simulink model "WS_3DRobot_example_V2"  (R2023a)
settings: Solver=ode2  StartTime=0.0  StopTime=tsim  FixedStep=t_sample  RelTol=1e-3
values from neighbouring files (symbols this model uses):
  initialConfig = homeConfiguration(robot)    [Indy4_Matlab_Robo_Code.m]    (also in simout.mat = [0 0 0 0 0 0])
  Kd1 = 10    [Indy4_Matlab_Robo_Code.m]    (also in simout.mat)
  Kd2 = 10    [Indy4_Matlab_Robo_Code.m]    (also in simout.mat)
  Kd3 = 10    [Indy4_Matlab_Robo_Code.m]    (also in simout.mat)
  Kfilt1 = 150    [Indy4_Matlab_Robo_Code.m]    (also in simout.mat)
  Kfilt2 = 150    [Indy4_Matlab_Robo_Code.m]    (also in simout.mat)
  Kfilt3 = 150    [Indy4_Matlab_Robo_Code.m]    (also in simout.mat)
  Kp1 = 100    [Indy4_Matlab_Robo_Code.m]    (also in simout.mat)
  Kp2 = 100    [Indy4_Matlab_Robo_Code.m]    (also in simout.mat)
  Kp3 = 100    [Indy4_Matlab_Robo_Code.m]    (also in simout.mat)
undefined symbols (not defined in the file or in its folder): ctrlLowerLimit, ctrlUpperLimit, eePos_des_sim, eul2tform
libraries: robotmaniplib x6, robotcorelib x4, slpidlib x3
settings Model: Creator=ha281  LastModifiedBy=james
settings SolverCC: AlgebraicLoopSolver=TrustRegion
settings DataIOCC: ReturnWorkspaceOutputs=off
settings DebuggingCC: UnconnectedInputMsg=warning  UnconnectedOutputMsg=warning  UnconnectedLineMsg=warning  ArithmeticOperatorsInVariantConditions=warning
settings ModelReferenceCC: EnableRefExpFcnMdlSchedulingChecks=on
settings SFSimCC: SimUseLocalCustomCode=off  CustomCodeUndefinedFunction=UseInterfaceOnly
settings RTWCC: RTWUseLocalCustomCode=off
settings CodeAppCC: StateflowObjectComments=on

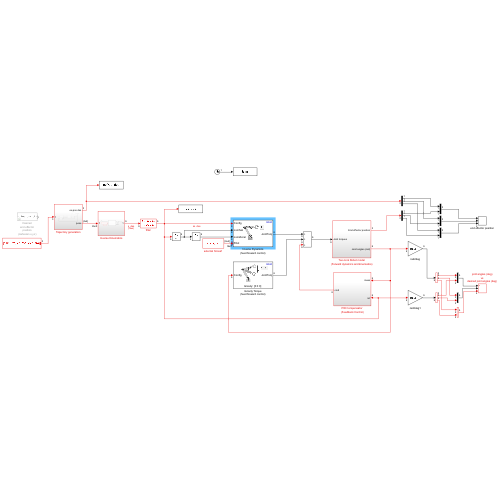
[thumbnail: Simulink's stored preview of the top-level diagram]
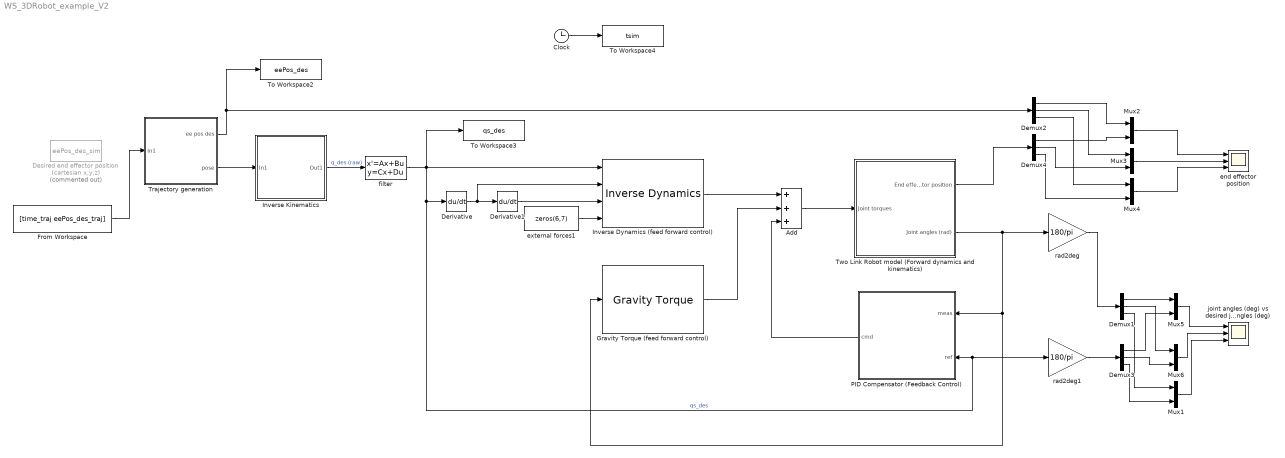
== system WS_3DRobot_example_V2 ==
  Add : Sum  Inputs=+++
  Clock : Clock
  Demux{1..4} (4 alike) : Demux  Outputs=3
  Derivative : Derivative
  Derivative1 : Derivative
  Desired end effector position (cartesian x,y,z) : Constant  Commented=on  Value=eePos_des_sim
  From Workspace : FromWorkspace  VariableName=[time_traj eePos_des_traj]
  Gravity Torque (feed forward control) : robotmaniplib/Gravity Torque  RigidBodyTree=robot  SimulateUsing=Interpreted execution
  Inverse Dynamics (feed forward control) : robotmaniplib/Inverse Dynamics  RigidBodyTree=robot  SimulateUsing=Interpreted execution
  Inverse Kinematics : Subsystem
  Mux{1..6} (6 alike) : Mux  Inputs=2
  PID Compensator (Feedback Control) : Subsystem
  To Workspace2 : ToWorkspace  VariableName=eePos_des  SampleTime=-1
  To Workspace3 : ToWorkspace  VariableName=qs_des  SampleTime=-1
  To Workspace4 : ToWorkspace  VariableName=tsim  SampleTime=-1
  Trajectory generation : Subsystem
  Two Link Robot model (Forward dynamics and kinematics) : Subsystem
  end effector position : Scope  NumInputPorts=3
  external forces1 : Constant  Value=zeros(6,7)
  filter : StateSpace  A=-1*eye(6)  B=1*eye(6)  C=eye(6)  D=zeros(6,6)  InitialCondition=0
  joint angles (deg) vs desired joint angles (deg) : Scope  NumInputPorts=3
  rad2deg : Gain  Gain=180/pi
  rad2deg1 : Gain  Gain=180/pi
  wires:
  Clock/1 -> To Workspace4/1
  rad2deg/1 -> Demux1/1
  Two Link Robot model (Forward dynamics and kinematics)/2(Joint angles (rad)) -> Gravity Torque (feed forward control)/1, PID Compensator (Feedback Control)/1(meas), rad2deg/1
  Derivative/1 -> Inverse Dynamics (feed forward control)/2, Derivative1/1
  Derivative1/1 -> Inverse Dynamics (feed forward control)/3
  external forces1/1 -> Inverse Dynamics (feed forward control)/4
  Inverse Dynamics (feed forward control)/1 -> Add/1
  Gravity Torque (feed forward control)/1 -> Add/2
  Add/1 -> Two Link Robot model (Forward dynamics and kinematics)/1(Joint torques)
  PID Compensator (Feedback Control)/1(cmd) -> Add/3
  Demux1/1 -> Mux5/1
  Demux3/2 -> Mux6/2
  Mux5/1 -> joint angles (deg) vs desired joint angles (deg)/1
  Demux3/1 -> Mux5/2
  Demux1/2 -> Mux6/1
  Mux6/1 -> joint angles (deg) vs desired joint angles (deg)/2
  rad2deg1/1 -> Demux3/1
  filter/1 -> To Workspace3/1, rad2deg1/1, PID Compensator (Feedback Control)/2(ref), Derivative/1, Inverse Dynamics (feed forward control)/1  "qs_des"
  Inverse Kinematics/1(Out1) -> filter/1  "q_des (raw)"
  Trajectory generation/2(pose) -> Inverse Kinematics/1(In1)
  Demux2/3 -> Mux4/1
  Trajectory generation/1(ee pos des) -> To Workspace2/1, Demux2/1
  Mux4/1 -> end effector position/3
  Demux4/3 -> Mux4/2
  Two Link Robot model (Forward dynamics and kinematics)/1(End effector position) -> Demux4/1
  Demux2/2 -> Mux3/1
  Mux3/1 -> end effector position/2
  Demux4/1 -> Mux2/2
  Mux2/1 -> end effector position/1
  Demux4/2 -> Mux3/2
  Demux2/1 -> Mux2/1
  From Workspace/1 -> Trajectory generation/1(In1)
  Demux1/3 -> Mux1/1
  Demux3/3 -> Mux1/2
  Mux1/1 -> joint angles (deg) vs desired joint angles (deg)/3

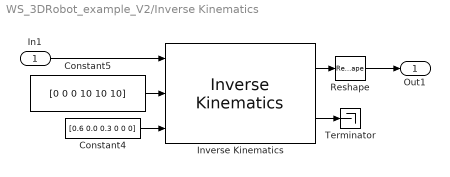
== system WS_3DRobot_example_V2/Inverse Kinematics ==
  In1 : Inport
  Constant4 : Constant  Value=[0.6 0.0 0.3 0 0 0]
  Constant5 : Constant  Value=[0 0 0 10 10 10]
  Inverse Kinematics : robotmaniplib/Inverse Kinematics  RigidBodyTree=robot  EndEffector=tool  ShowInfo=on  SolverName=BFGS Gradient Projection  EnforceJointLimits=on  MaxIterations=1500  MaxTime=10  GradientTolerance=1e-7  SolutionTolerance=1e-6  StepTolerance=1e-14  ErrorChangeTolerance=1e-12  UseErrorDamping=on  DampingBias=0.0025  SimulateUsing=Interpreted execution
  Reshape : Reshape
  Terminator : Terminator
  Out1 : Outport
  wires:
  Constant5/1 -> Inverse Kinematics/2
  Inverse Kinematics/2 -> Terminator/1
  Inverse Kinematics/1 -> Reshape/1
  Constant4/1 -> Inverse Kinematics/3
  Reshape/1 -> Out1/1
  In1/1 -> Inverse Kinematics/1

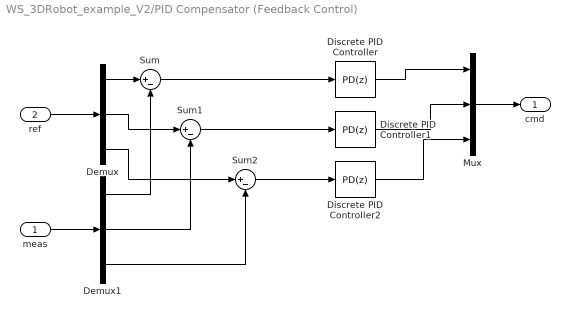
== system WS_3DRobot_example_V2/PID Compensator (Feedback Control) ==
  meas : Inport
  ref : Inport  Port=2
  Demux : Demux  Outputs=3
  Demux1 : Demux  Outputs=3
  Discrete PID Controller : slpidlib/PID Controller  Controller=PD  Form=Parallel  TimeDomain=Discrete-time  UseExternalTs=off  SampleTime=-1  IntegratorMethod=Forward Euler  FilterMethod=Forward Euler  ControllerParametersSource=internal  P=Kp1  I=0.01  UseKiTs=off  D=Kd1  N=Kfilt1  UseFilter=on  TunerSelectOption=Transfer Function Based (PID Tuner App)  InitialConditionSource=internal  InitialConditionForIntegrator=0  InitialConditionForFilter=0  DifferentiatorICPrevScaledInput=0  ExternalReset=none  TrackingMode=off  Kt=1  LimitOutput=off  SatLimitsSource=internal  UpperSaturationLimit=ctrlUpperLimit  LowerSaturationLimit=ctrlLowerLimit  LinearizeAsGain=off  AntiWindupMode=clamping  Kb=1  LimitIntegrator=off  UpperIntegratorSaturationLimit=inf  LowerIntegratorSaturationLimit=-inf  POutMin=[]  POutMax=[]  IOutMin=[]  IOutMax=[]  DOutMin=[]  DOutMax=[]  NOutMin=[]  NOutMax=[]  SumOutMin=[]  SumOutMax=[]  SaturationOutMin=[]  SaturationOutMax=[]  PParamMin=[]  PParamMax=[]  IParamMin=[]  IParamMax=[]  DParamMin=[]  DParamMax=[]  NParamMin=[]  NParamMax=[]  KbParamMin=[]  KbParamMax=[]  KtParamMin=[]  KtParamMax=[]  KbOutMin=[]  KbOutMax=[]  KtOutMin=[]  KtOutMax=[]  IntegratorOutMin=[]  IntegratorOutMax=[]  FilterOutMin=[]  FilterOutMax=[]  SumI1OutMin=[]  SumI1OutMax=[]  SumI2OutMin=[]  SumI2OutMax=[]  SumI3OutMin=[]  SumI3OutMax=[]  SumI4OutMin=[]  SumI4OutMax=[]  SumDOutMin=[]  SumDOutMax=[]  DifferentiatorOutMin=[]  DifferentiatorOutMax=[]  FilterDiffOutCoefMin=[]  FilterDiffOutCoefMax=[]  ReciprocalOutMin=[]  ReciprocalOutMax=[]  SumDenOutMin=[]  SumDenOutMax=[]  SumNumOutMin=[]  SumNumOutMax=[]  DivideOutMin=[]  DivideOutMax=[]  UdiffTsProdOutMin=[]  UdiffTsProdOutMax=[]  NTsProdOutMin=[]  NTsProdOutMax=[]  UintegralTsProdOutMin=[]  UintegralTsProdOutMax=[]  UngainTsProdOutMin=[]  UngainTsProdOutMax=[]  ClampingZeroOutDataTypeStr=Inherit: Inherit via back propagation  ClampingZeroOutMin=[]  ClampingZeroOutMax=[]  FilterDenConstantOutDataTypeStr=Inherit: Inherit via back propagation  FilterDenConstantOutMin=[]  FilterDenConstantOutMax=[]  PCopyOutDataTypeStr=Inherit: Inherit via back propagation  PCopyOutMin=[]  PCopyOutMax=[]  NCopyOutDataTypeStr=Inherit: Inherit via back propagation  NCopyOutMin=[]  NCopyOutMax=[]  IntegratorContinuousStateAttributes=''  IntegratorStateMustResolveToSignalObject=off  IntegratorRTWStateStorageClass=Auto  FilterContinuousStateAttributes=''  FilterStateMustResolveToSignalObject=off  FilterRTWStateStorageClass=Auto  ParallelPVariant=InternalParameters  IdealPVariant=Disabled  IVariant=Disabled  DVariant=InternalParameters  IntegratorVariant=Disabled  SatVariant=Disabled  AWVariant=Disabled  PCopyVariant=Disabled  TRVariant=Disabled  FdbkBlocksVariant=Forward  IdealPFdbkVariant=Disabled  SatFdbkVariant=Disabled  DerivativeFilterVariant=ForwardEulerFilter  NVariant=InternalParameters  NCopyVariant=Disabled  FilterICVariant=InternalICsFilter  IntegratorICVariant=Disabled  ExternalResetVariant=Disabled  TRSumVariant=Passthrough  SumFdbkVariant=Disabled  SumVariant=Sum_PD  TsampFilterVariant=InternalTs  TsampNgainVariant=Passthrough  TsampIntegralVariant=Disabled_SignalSpec  ExternalSaturationOutDataTypeStr=Inherit: Same as second input
  Discrete PID Controller1 : slpidlib/PID Controller  Controller=PD  Form=Parallel  TimeDomain=Discrete-time  UseExternalTs=off  SampleTime=-1  IntegratorMethod=Forward Euler  FilterMethod=Forward Euler  ControllerParametersSource=internal  P=Kp2  I=0.01  UseKiTs=off  D=Kd2  N=Kfilt2  UseFilter=on  TunerSelectOption=Transfer Function Based (PID Tuner App)  InitialConditionSource=internal  InitialConditionForIntegrator=0  InitialConditionForFilter=0  DifferentiatorICPrevScaledInput=0  ExternalReset=none  TrackingMode=off  Kt=1  LimitOutput=off  SatLimitsSource=internal  UpperSaturationLimit=ctrlUpperLimit  LowerSaturationLimit=ctrlLowerLimit  LinearizeAsGain=off  AntiWindupMode=clamping  Kb=1  LimitIntegrator=off  UpperIntegratorSaturationLimit=inf  LowerIntegratorSaturationLimit=-inf  POutMin=[]  POutMax=[]  IOutMin=[]  IOutMax=[]  DOutMin=[]  DOutMax=[]  NOutMin=[]  NOutMax=[]  SumOutMin=[]  SumOutMax=[]  SaturationOutMin=[]  SaturationOutMax=[]  PParamMin=[]  PParamMax=[]  IParamMin=[]  IParamMax=[]  DParamMin=[]  DParamMax=[]  NParamMin=[]  NParamMax=[]  KbParamMin=[]  KbParamMax=[]  KtParamMin=[]  KtParamMax=[]  KbOutMin=[]  KbOutMax=[]  KtOutMin=[]  KtOutMax=[]  IntegratorOutMin=[]  IntegratorOutMax=[]  FilterOutMin=[]  FilterOutMax=[]  SumI1OutMin=[]  SumI1OutMax=[]  SumI2OutMin=[]  SumI2OutMax=[]  SumI3OutMin=[]  SumI3OutMax=[]  SumI4OutMin=[]  SumI4OutMax=[]  SumDOutMin=[]  SumDOutMax=[]  DifferentiatorOutMin=[]  DifferentiatorOutMax=[]  FilterDiffOutCoefMin=[]  FilterDiffOutCoefMax=[]  ReciprocalOutMin=[]  ReciprocalOutMax=[]  SumDenOutMin=[]  SumDenOutMax=[]  SumNumOutMin=[]  SumNumOutMax=[]  DivideOutMin=[]  DivideOutMax=[]  UdiffTsProdOutMin=[]  UdiffTsProdOutMax=[]  NTsProdOutMin=[]  NTsProdOutMax=[]  UintegralTsProdOutMin=[]  UintegralTsProdOutMax=[]  UngainTsProdOutMin=[]  UngainTsProdOutMax=[]  ClampingZeroOutDataTypeStr=Inherit: Inherit via back propagation  ClampingZeroOutMin=[]  ClampingZeroOutMax=[]  FilterDenConstantOutDataTypeStr=Inherit: Inherit via back propagation  FilterDenConstantOutMin=[]  FilterDenConstantOutMax=[]  PCopyOutDataTypeStr=Inherit: Inherit via back propagation  PCopyOutMin=[]  PCopyOutMax=[]  NCopyOutDataTypeStr=Inherit: Inherit via back propagation  NCopyOutMin=[]  NCopyOutMax=[]  IntegratorContinuousStateAttributes=''  IntegratorStateMustResolveToSignalObject=off  IntegratorRTWStateStorageClass=Auto  FilterContinuousStateAttributes=''  FilterStateMustResolveToSignalObject=off  FilterRTWStateStorageClass=Auto  ParallelPVariant=InternalParameters  IdealPVariant=Disabled  IVariant=Disabled  DVariant=InternalParameters  IntegratorVariant=Disabled  SatVariant=Disabled  AWVariant=Disabled  PCopyVariant=Disabled  TRVariant=Disabled  FdbkBlocksVariant=Forward  IdealPFdbkVariant=Disabled  SatFdbkVariant=Disabled  DerivativeFilterVariant=ForwardEulerFilter  NVariant=InternalParameters  NCopyVariant=Disabled  FilterICVariant=InternalICsFilter  IntegratorICVariant=Disabled  ExternalResetVariant=Disabled  TRSumVariant=Passthrough  SumFdbkVariant=Disabled  SumVariant=Sum_PD  TsampFilterVariant=InternalTs  TsampNgainVariant=Passthrough  TsampIntegralVariant=Disabled_SignalSpec  ExternalSaturationOutDataTypeStr=Inherit: Same as second input
  Discrete PID Controller2 : slpidlib/PID Controller  Controller=PD  Form=Parallel  TimeDomain=Discrete-time  UseExternalTs=off  SampleTime=-1  IntegratorMethod=Forward Euler  FilterMethod=Forward Euler  ControllerParametersSource=internal  P=Kp3  I=0.01  UseKiTs=off  D=Kd3  N=Kfilt3  UseFilter=on  TunerSelectOption=Transfer Function Based (PID Tuner App)  InitialConditionSource=internal  InitialConditionForIntegrator=0  InitialConditionForFilter=0  DifferentiatorICPrevScaledInput=0  ExternalReset=none  TrackingMode=off  Kt=1  LimitOutput=off  SatLimitsSource=internal  UpperSaturationLimit=ctrlUpperLimit  LowerSaturationLimit=ctrlLowerLimit  LinearizeAsGain=off  AntiWindupMode=clamping  Kb=1  LimitIntegrator=off  UpperIntegratorSaturationLimit=inf  LowerIntegratorSaturationLimit=-inf  POutMin=[]  POutMax=[]  IOutMin=[]  IOutMax=[]  DOutMin=[]  DOutMax=[]  NOutMin=[]  NOutMax=[]  SumOutMin=[]  SumOutMax=[]  SaturationOutMin=[]  SaturationOutMax=[]  PParamMin=[]  PParamMax=[]  IParamMin=[]  IParamMax=[]  DParamMin=[]  DParamMax=[]  NParamMin=[]  NParamMax=[]  KbParamMin=[]  KbParamMax=[]  KtParamMin=[]  KtParamMax=[]  KbOutMin=[]  KbOutMax=[]  KtOutMin=[]  KtOutMax=[]  IntegratorOutMin=[]  IntegratorOutMax=[]  FilterOutMin=[]  FilterOutMax=[]  SumI1OutMin=[]  SumI1OutMax=[]  SumI2OutMin=[]  SumI2OutMax=[]  SumI3OutMin=[]  SumI3OutMax=[]  SumI4OutMin=[]  SumI4OutMax=[]  SumDOutMin=[]  SumDOutMax=[]  DifferentiatorOutMin=[]  DifferentiatorOutMax=[]  FilterDiffOutCoefMin=[]  FilterDiffOutCoefMax=[]  ReciprocalOutMin=[]  ReciprocalOutMax=[]  SumDenOutMin=[]  SumDenOutMax=[]  SumNumOutMin=[]  SumNumOutMax=[]  DivideOutMin=[]  DivideOutMax=[]  UdiffTsProdOutMin=[]  UdiffTsProdOutMax=[]  NTsProdOutMin=[]  NTsProdOutMax=[]  UintegralTsProdOutMin=[]  UintegralTsProdOutMax=[]  UngainTsProdOutMin=[]  UngainTsProdOutMax=[]  ClampingZeroOutDataTypeStr=Inherit: Inherit via back propagation  ClampingZeroOutMin=[]  ClampingZeroOutMax=[]  FilterDenConstantOutDataTypeStr=Inherit: Inherit via back propagation  FilterDenConstantOutMin=[]  FilterDenConstantOutMax=[]  PCopyOutDataTypeStr=Inherit: Inherit via back propagation  PCopyOutMin=[]  PCopyOutMax=[]  NCopyOutDataTypeStr=Inherit: Inherit via back propagation  NCopyOutMin=[]  NCopyOutMax=[]  IntegratorContinuousStateAttributes=''  IntegratorStateMustResolveToSignalObject=off  IntegratorRTWStateStorageClass=Auto  FilterContinuousStateAttributes=''  FilterStateMustResolveToSignalObject=off  FilterRTWStateStorageClass=Auto  ParallelPVariant=InternalParameters  IdealPVariant=Disabled  IVariant=Disabled  DVariant=InternalParameters  IntegratorVariant=Disabled  SatVariant=Disabled  AWVariant=Disabled  PCopyVariant=Disabled  TRVariant=Disabled  FdbkBlocksVariant=Forward  IdealPFdbkVariant=Disabled  SatFdbkVariant=Disabled  DerivativeFilterVariant=ForwardEulerFilter  NVariant=InternalParameters  NCopyVariant=Disabled  FilterICVariant=InternalICsFilter  IntegratorICVariant=Disabled  ExternalResetVariant=Disabled  TRSumVariant=Passthrough  SumFdbkVariant=Disabled  SumVariant=Sum_PD  TsampFilterVariant=InternalTs  TsampNgainVariant=Passthrough  TsampIntegralVariant=Disabled_SignalSpec  ExternalSaturationOutDataTypeStr=Inherit: Same as second input
  Mux : Mux  Inputs=3
  Sum : Sum  Inputs=|+-
  Sum1 : Sum  Inputs=|+-
  Sum2 : Sum  Inputs=|+-
  cmd : Outport  VectorParamsAs1DForOutWhenUnconnected=off
  wires:
  Demux1/2 -> Sum1/2
  Discrete PID Controller1/1 -> Mux/2
  Demux/2 -> Sum1/1
  Sum1/1 -> Discrete PID Controller1/1
  Mux/1 -> cmd/1
  Discrete PID Controller/1 -> Mux/1
  Sum/1 -> Discrete PID Controller/1
  Demux1/1 -> Sum/2
  Demux/1 -> Sum/1
  meas/1 -> Demux1/1
  ref/1 -> Demux/1
  Demux/3 -> Sum2/1
  Demux1/3 -> Sum2/2
  Sum2/1 -> Discrete PID Controller2/1
  Discrete PID Controller2/1 -> Mux/3

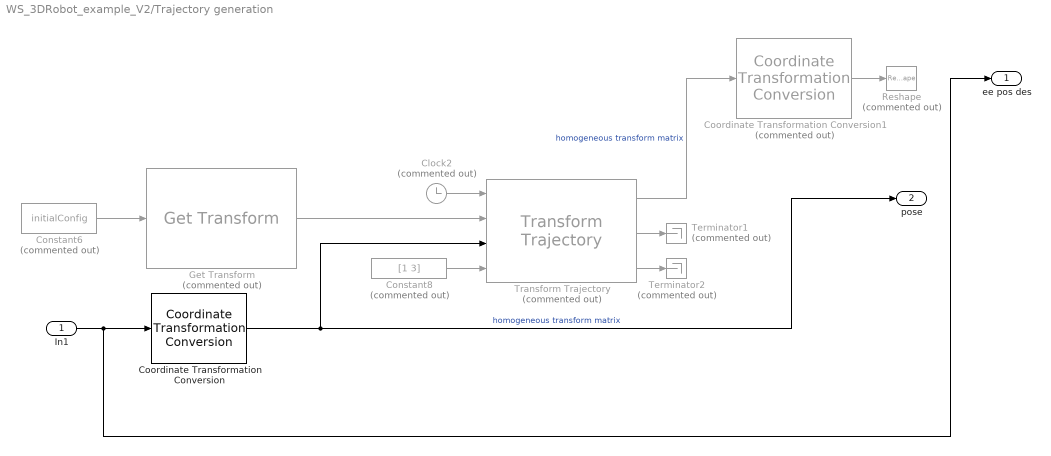
== system WS_3DRobot_example_V2/Trajectory generation ==
  In1 : Inport
  Clock2 : Clock  Commented=on
  Constant6 : Constant  Commented=on  Value=initialConfig
  Constant8 : Constant  Commented=on  Value=[1 3]
  Coordinate Transformation Conversion : robotcorelib/Coordinate Transformation Conversion  InputRepresentation=Translation Vector  InputEulerSequence=ZYX  ShowTrVecInputPort=on  OutputRepresentation=Homogeneous Transformation  OutputEulerSequence=ZYX  ShowTrVecOutputPort=on  SimulateUsing=Interpreted execution
  Coordinate Transformation Conversion1 : robotcorelib/Coordinate Transformation Conversion  Commented=on  InputRepresentation=Homogeneous Transformation  InputEulerSequence=ZYX  ShowTrVecInputPort=on  OutputRepresentation=Translation Vector  OutputEulerSequence=ZYX  ShowTrVecOutputPort=on  SimulateUsing=Interpreted execution
  Get Transform : robotmaniplib/Get Transform  Commented=on  RigidBodyTree=robot  SourceBody=tool  TargetBody=base  SimulateUsing=Interpreted execution
  Reshape : Reshape  Commented=on
  Terminator1 : Terminator  Commented=on
  Terminator2 : Terminator  Commented=on
  Transform Trajectory : robotcorelib/Transform Trajectory  Commented=on  WaypointSource=External  T0=eul2tform( [ 0.6, 0, 0 ] )  TF=eul2tform( [ 0.45, 0.1, 0 ] )  TimeInterval=[ 2, 3 ]  CustomTimeScaling=off  ParameterSource=Internal  TSTime=2:0.1:3  TimeScaling=[ 0:0.1:1; ones( 1, 11 ); zeros( 1, 11 ) ]  SimulateUsing=Interpreted execution
  ee pos des : Outport
  pose : Outport  Port=2
  wires:
  Get Transform/1 -> Transform Trajectory/2
  Constant6/1 -> Get Transform/1
  Coordinate Transformation Conversion/1 -> pose/1, Transform Trajectory/3  "homogeneous transform matrix"
  Clock2/1 -> Transform Trajectory/1
  Transform Trajectory/2 -> Terminator1/1
  Constant8/1 -> Transform Trajectory/4
  Transform Trajectory/3 -> Terminator2/1
  In1/1 -> ee pos des/1, Coordinate Transformation Conversion/1
  Coordinate Transformation Conversion1/1 -> Reshape/1
  Transform Trajectory/1 -> Coordinate Transformation Conversion1/1  "homogeneous transform matrix"

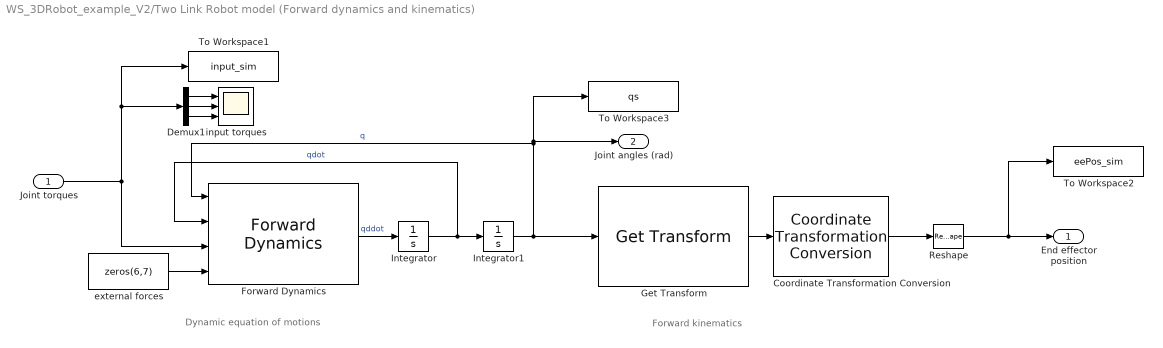
== system WS_3DRobot_example_V2/Two Link Robot model (Forward dynamics and kinematics) ==
  note: Forward kinematics
  note: Dynamic equation of motions
  Joint torques : Inport
  Coordinate Transformation Conversion : robotcorelib/Coordinate Transformation Conversion  InputRepresentation=Homogeneous Transformation  InputEulerSequence=ZYX  ShowTrVecInputPort=on  OutputRepresentation=Translation Vector  OutputEulerSequence=ZYX  ShowTrVecOutputPort=on  SimulateUsing=Interpreted execution
  Demux1 : Demux  Outputs=3
  Forward Dynamics : robotmaniplib/Forward Dynamics  RigidBodyTree=robot  SimulateUsing=Interpreted execution
  Get Transform : robotmaniplib/Get Transform  RigidBodyTree=robot  SourceBody=tool  TargetBody=base  SimulateUsing=Interpreted execution
  Integrator : Integrator
  Integrator1 : Integrator
  Reshape : Reshape
  To Workspace1 : ToWorkspace  VariableName=input_sim  SampleTime=-1
  To Workspace2 : ToWorkspace  VariableName=eePos_sim  SampleTime=-1
  To Workspace3 : ToWorkspace  VariableName=qs  SampleTime=-1
  external forces : Constant  Value=zeros(6,7)
  input torques : Scope  NumInputPorts=3
  End effector position : Outport
  Joint angles (rad) : Outport  Port=2
  wires:
  Integrator/1 -> Forward Dynamics/2, Integrator1/1  "qdot"
  Forward Dynamics/1 -> Integrator/1  "qddot"
  Demux1/2 -> input torques/2
  external forces/1 -> Forward Dynamics/4
  Reshape/1 -> End effector position/1, To Workspace2/1
  Integrator1/1 -> Get Transform/1, To Workspace3/1, Joint angles (rad)/1, Forward Dynamics/1  "q"
  Joint torques/1 -> Demux1/1, To Workspace1/1, Forward Dynamics/3
  Get Transform/1 -> Coordinate Transformation Conversion/1
  Demux1/1 -> input torques/1
  Coordinate Transformation Conversion/1 -> Reshape/1
  Demux1/3 -> input torques/3
